simulink model "Linear_model"  (R2025b)
settings: Solver=VariableStepAuto  StartTime=0.0  StopTime=20  RelTol=1e-3
values from neighbouring files (symbols this model uses):
  A1 = [0, 1; 0, 0]    [linear_validation.m]
  A2 = [0, 0, 1, 0; 0, 0, 0, 1; 0, g, 0, 0; 0, 0, 0, 0]    [linear_validation.m]
  A3 = [0, 0, 1, 0; 0, 0, 0, 1; 0, -g, 0, 0; 0, 0, 0, 0]    [linear_validation.m]
  A4 = [0, 1; 0, 0]    [linear_validation.m]
  B1 = [0; 1/m]    [linear_validation.m]
  B2 = [0; 0; 0; 1/J11]    [linear_validation.m]
  B3 = [0; 0; 0; 1/J22]    [linear_validation.m]
  B4 = [0; 1/J33]    [linear_validation.m]
  C1 = eye(2)    [linear_validation.m]
  C2 = eye(4)    [linear_validation.m]
  C3 = eye(4)    [linear_validation.m]
  C4 = eye(2)    [linear_validation.m]
  D1 = zeros(2,1)    [linear_validation.m]
  D2 = zeros(4,1)    [linear_validation.m]
  D3 = zeros(4,1)    [linear_validation.m]
  D4 = zeros(2,1)    [linear_validation.m]
  g = 9.81    [drone_model_parameters.mat]
  J11 = 5.8286e-05    [drone_model_parameters.mat]
  J22 = 7.1691e-05    [drone_model_parameters.mat]
  J33 = 3e-05    [drone_model_parameters.mat]
  K_T = 4.72e-08    [drone_model_parameters.mat]
  K_tau = 1.1393e-10    [drone_model_parameters.mat]
  K_u = 13840.4    [drone_model_parameters.mat]
  L = 0.0624    [drone_model_parameters.mat]
  m = 0.063    [drone_model_parameters.mat]
  u_imax = 500    [drone_model_parameters.mat]
settings Model: Creator=Lenovo  LastModifiedBy=pepev

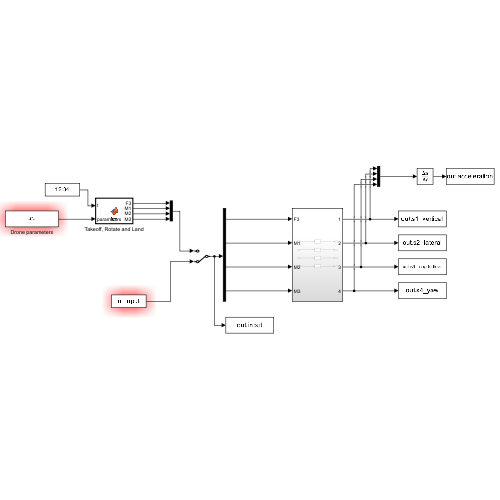
[thumbnail: Simulink's stored preview of the top-level diagram]
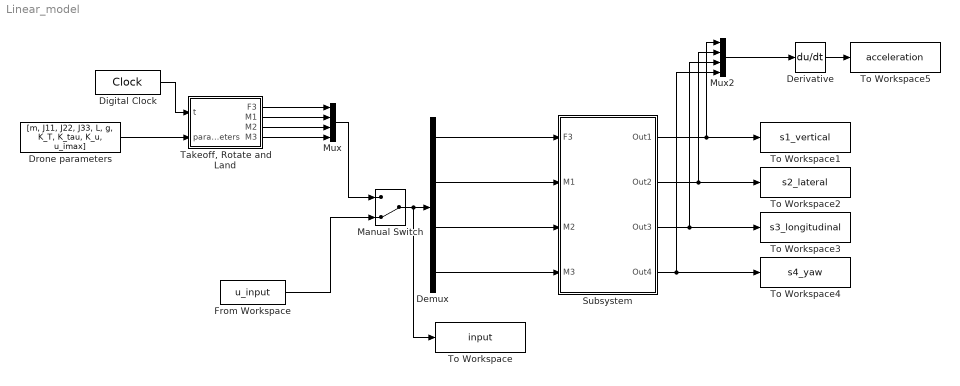
== system Linear_model ==
  Demux : Demux
  Derivative : Derivative
  Digital Clock : DigitalClock  SampleTime=0.01
  Drone parameters : Constant  Value=[m, J11, J22, J33, L, g, K_T, K_tau, K_u, u_imax]
  From Workspace : FromWorkspace  VariableName=u_input
  Manual Switch : ManualSwitch  CurrentSetting=0
  Mux : Mux
  Mux2 : Mux
  Subsystem : Subsystem
  "Takeoff, Rotate and Land" : MATLAB Function  TreatAsAtomicUnit=on
  To Workspace : ToWorkspace  VariableName=input  SaveFormat=Timeseries  SampleTime=-1
  To Workspace1 : ToWorkspace  VariableName=s1_vertical  SaveFormat=Timeseries  SampleTime=-1
  To Workspace2 : ToWorkspace  VariableName=s2_lateral  SaveFormat=Timeseries  SampleTime=-1
  To Workspace3 : ToWorkspace  VariableName=s3_longitudinal  SaveFormat=Timeseries  SampleTime=-1
  To Workspace4 : ToWorkspace  VariableName=s4_yaw  SaveFormat=Timeseries  SampleTime=-1
  To Workspace5 : ToWorkspace  VariableName=acceleration  SaveFormat=Timeseries  SampleTime=-1
  wires:
  Subsystem/1(Out1) -> To Workspace1/1, Mux2/1
  Subsystem/2(Out2) -> To Workspace2/1, Mux2/2
  Subsystem/3(Out3) -> To Workspace3/1, Mux2/3
  Subsystem/4(Out4) -> Mux2/4, To Workspace4/1
  Digital Clock/1 -> "Takeoff, Rotate and Land"/1(t)
  Drone parameters/1 -> "Takeoff, Rotate and Land"/2(parameters)
  "Takeoff, Rotate and Land"/1(F3) -> Mux/1
  "Takeoff, Rotate and Land"/2(M1) -> Mux/2
  "Takeoff, Rotate and Land"/3(M2) -> Mux/3
  "Takeoff, Rotate and Land"/4(M3) -> Mux/4
  Mux/1 -> Manual Switch/1
  Manual Switch/1 -> To Workspace/1, Demux/1
  Demux/4 -> Subsystem/4(M3)
  Demux/3 -> Subsystem/3(M2)
  Demux/2 -> Subsystem/2(M1)
  Demux/1 -> Subsystem/1(F3)
  Mux2/1 -> Derivative/1
  Derivative/1 -> To Workspace5/1
  From Workspace/1 -> Manual Switch/2

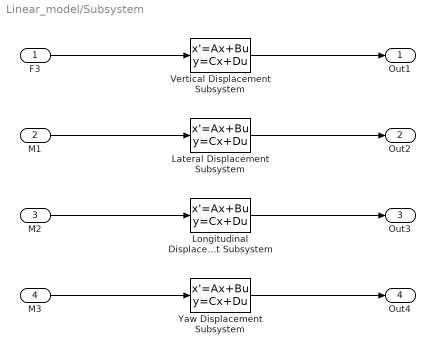
== system Linear_model/Subsystem ==
  F3 : Inport
  M1 : Inport  Port=2
  M2 : Inport  Port=3
  M3 : Inport  Port=4
  Lateral Displacement Subsystem : StateSpace  A=A2  B=B2  C=C2  D=D2  InitialCondition=0
  Longitudinal Displacement Subsystem : StateSpace  A=A3  B=B3  C=C3  D=D3  InitialCondition=0
  Vertical Displacement Subsystem : StateSpace  A=A1  B=B1  C=C1  D=D1  InitialCondition=0
  Yaw Displacement Subsystem : StateSpace  A=A4  B=B4  C=C4  D=D4  InitialCondition=0
  Out1 : Outport
  Out2 : Outport  Port=2
  Out3 : Outport  Port=3
  Out4 : Outport  Port=4
  wires:
  F3/1 -> Vertical Displacement Subsystem/1
  Vertical Displacement Subsystem/1 -> Out1/1
  M1/1 -> Lateral Displacement Subsystem/1
  M2/1 -> Longitudinal Displacement Subsystem/1
  M3/1 -> Yaw Displacement Subsystem/1
  Lateral Displacement Subsystem/1 -> Out2/1
  Longitudinal Displacement Subsystem/1 -> Out3/1
  Yaw Displacement Subsystem/1 -> Out4/1

== matlab function Linear_model/Takeoff, Rotate and Land ==
  data: t input; F3 output; parameters input; M1 output; M2 output; M3 output
function [F3,M1,M2,M3] = fcn(t, parameters)
% ── Trajectory generation for the LINEAR quadcopter model ────────────────
% Computes the control inputs (F3, M1, M2, M3) at each time instant t
% for a Takeoff → Rotate → Land maneuver.
%
% Inputs:
%   t          - current simulation time [s]
%   parameters - drone parameter vector [m, J11, J22, J33, ?, g]
%
% Outputs:
%   F3  - vertical thrust perturbation [N]   (deviation from hover)
%   M1  - roll moment [N·m]                  (zero throughout)
%   M2  - pitch moment [N·m]                 (zero throughout)
%   M3  - yaw moment [N·m]

    % ── Extract parameters ────────────────────────────────────────────────
    m   = parameters(1);   % drone mass [kg]
    J33 = parameters(4);   % yaw moment of inertia [kg·m²]

    % ── Maneuver timing ───────────────────────────────────────────────────
    t_to   = 5;    % takeoff duration [s]
    t_rot  = 10;   % rotation duration [s]
    t_land = 5;    % landing duration [s]

    % ── Acceleration amplitudes (from Eq. 2.23) ───────────────────────────
    alfa_to   = -0.016;   % takeoff vertical acceleration [m/s²]
    alfa_rot  =  pi/25;   % yaw angular acceleration [rad/s²]
    alfa_land =  0.016;   % landing vertical acceleration [m/s²]

    % ── Piecewise acceleration profile (Eq. 2.23) ─────────────────────────
    % Generates a trapezoidal velocity profile over duration tf:
    %   first  half [0,    tf/2]: constant +alfa  (accelerate)
    %   second half [tf/2, tf]:   constant -alfa  (decelerate)
    %   outside [0, tf]:          zero            (no motion)
    function q_ddot = acceleration(alfa, tf, t)
        if t >= 0 && t < tf/2
            q_ddot = alfa;       % acceleration phase
        elseif t >= tf/2 && t <= tf
            q_ddot = -alfa;      % deceleration phase
        else
            q_ddot = 0;          % outside maneuver window
        end
    end

    % ── Vertical thrust F3 ────────────────────────────────────────────────
    % Sum of takeoff and landing acceleration contributions.
    % Landing clock starts after takeoff + rotation are complete (t - t_to - t_rot).
    % Note: no -m*g term here because the linear model is linearized around
    % hover equilibrium — gravity is already accounted for at the operating point.
    F3 = m * acceleration(alfa_to,   t_to,   t) + ...
         m * acceleration(alfa_land, t_land, t - t_to - t_rot);

    % ── Roll and pitch moments ────────────────────────────────────────────
    % No lateral motion commanded — drone moves only vertically and in yaw.
    M1 = 0;
    M2 = 0;

    % ── Yaw moment M3 ─────────────────────────────────────────────────────
    % Rotation starts after takeoff is complete (t - t_to).
    M3 = J33 * acceleration(alfa_rot, t_rot, t - t_to);

end
